simulink model "remote_IAI_rcp"  (R2023a)
settings: Solver=ode1  StartTime=0.0  StopTime=inf  FixedStep=0.02  RelTol=1e-3
undefined symbols (not defined in the file): f, none, videoinput
libraries: simulink x9, instrumentlib x3, imaqlib x1, visionsinks x1
settings Model: Creator=nkobayas  LastModifiedBy=nkobayas

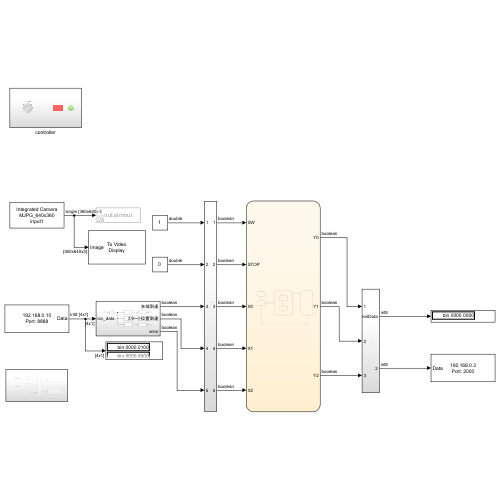
[thumbnail: Simulink's stored preview of the top-level diagram]
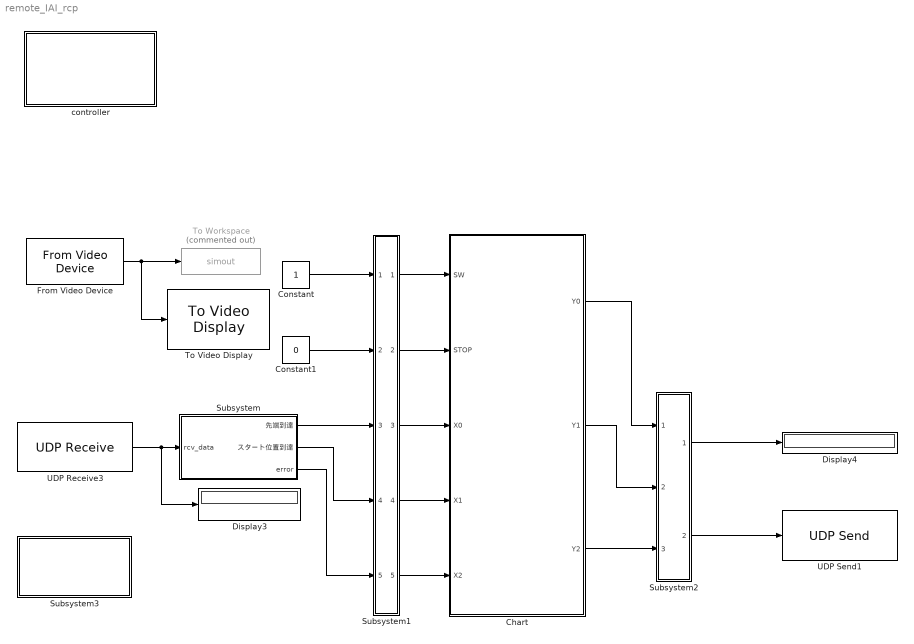
== system remote_IAI_rcp ==
  Chart : Stateflow chart  TreatAsAtomicUnit=on
  Constant : Constant
  Constant1 : Constant  Value=0
  Display3 : Display
      settings: Format=binary (Stored Integer)
  Display4 : Display
      settings: Format=binary (Stored Integer)
  From Video Device : imaqlib/From Video Device  DeviceMenu=winvideo 1 (Integrated Camera)  Device=winvideo 1 (Integrated Camera)  ObjConstructor=videoinput('winvideo', 1)  VideoFormatMenu=MJPG_640x360  VideoFormat=MJPG_640x360  VideoSource=input1  ROIPosition=[0 0 360 640]  EnableHWTrigger=off  TriggerConfiguration=none/none  SampleTime=0.02  OutputPortsMode=One multidimensional signal  DataType=single  CanDoHWTrigger=no  ReturnedColorSpace=rgb  BlockHandle=264.0006  ROIWidth=640  ROIHeight=360  ROIColumn=0  ROIRow=0  EngXMLPath=C:\Program Files\MATLAB\R2023a\toolbox\imaq\imaq\private  DevXMLPath=C:\ProgramData\MATLAB\SupportPackages\R2023a\toolbox\imaq\supportpackages\genericvideo\adaptor\win64  EngLibPath=C:\Program Files\MATLAB\R2023a\toolbox\imaq\imaqblks\imaqmex\win64  ColorSpace=rgb  BayerSensorAlignment=grbg  ImaqMode=off
  Subsystem : Subsystem
  Subsystem1 : Subsystem
  Subsystem2 : Subsystem
  Subsystem3 : Subsystem
  To Video Display : visionsinks/To Video Display  windowSizeMode=Normal  openAtMdlStart=on  fullScreen=off  videoWindowX=26  videoWindowY=640  saveWindowSize=off  videoWindowWidth=640  videoWindowHeight=360  inputColorFormat=RGB  inputType=Obsolete  imagePorts=One multidimensional signal  OutputDevice=On-screen video monitor  dataOrg=Column-major  isWindowOpen=off
  To Workspace : ToWorkspace  Commented=on  VariableName=simout  SaveFormat=Timeseries  SampleTime=-1
  UDP Receive3 : instrumentlib/UDP Receive  LocalAddress=192.168.0.10  LocalPort=8888  EnablePortSharing=on  Host=192.168.0.3  Port=2000  GetLatestData=on  DataSize=4  DataType=int8  ASCIIFormatting=%f,  Terminator=LF  CustomTerminator=10  ByteOrder=little-endian  EnableBlockingMode=on  Timeout=10  SampleTime=0.02  SimulateUsing=Interpreted execution
  UDP Send1 : instrumentlib/UDP Send  Host=192.168.0.3  Port=2000  LocalAddress=192.168.0.10  LocalPort=8888  EnablePortSharing=on  OutputDatagramPacketSize=8  ByteOrder=little-endian  EnableBlockingMode=off  SimulateUsing=Interpreted execution
  controller : Subsystem
  wires:
  Chart/3(Y2) -> Subsystem2/3(In3)
  Chart/2(Y1) -> Subsystem2/2(In2)
  Chart/1(Y0) -> Subsystem2/1(In1)
  Subsystem2/2(Out2) -> UDP Send1/1
  Subsystem2/1(serverSendData) -> Display4/1
  UDP Receive3/1 -> Subsystem/1(rcv_data), Display3/1
  Constant/1 -> Subsystem1/1(In1)
  Constant1/1 -> Subsystem1/2(In2)
  Subsystem/1(先端到達) -> Subsystem1/3(In3)
  Subsystem/2(スタート位置到達) -> Subsystem1/4(In4)
  Subsystem/3(error) -> Subsystem1/5(In5)
  Subsystem1/1(Out1) -> Chart/1(SW)
  Subsystem1/2(Out2) -> Chart/2(STOP)
  Subsystem1/3(Out3) -> Chart/3(X0)
  Subsystem1/4(Out4) -> Chart/4(X1)
  Subsystem1/5(Out5) -> Chart/5(X2)
  From Video Device/1 -> To Video Display/1, To Workspace/1

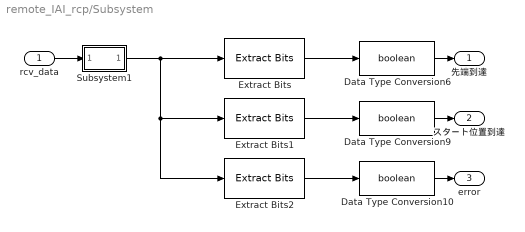
== system remote_IAI_rcp/Subsystem ==
  rcv_data : Inport
  Data Type Conversion10 : DataTypeConversion  OutDataTypeStr=boolean  SaturateOnIntegerOverflow=off  RndMeth=Floor
  Data Type Conversion6 : DataTypeConversion  OutDataTypeStr=boolean  SaturateOnIntegerOverflow=off  RndMeth=Floor
  Data Type Conversion9 : DataTypeConversion  OutDataTypeStr=boolean  SaturateOnIntegerOverflow=off  RndMeth=Floor
  Extract Bits : simulink/Logic and Bit Operations/Extract Bits  bitsToExtract=Range of bits  numBits=8  bitIdxRange=2  outScalingMode=Treat bit field as an integer
  Extract Bits1 : simulink/Logic and Bit Operations/Extract Bits  bitsToExtract=Range of bits  numBits=8  bitIdxRange=0  outScalingMode=Treat bit field as an integer
  Extract Bits2 : simulink/Logic and Bit Operations/Extract Bits  bitsToExtract=Range of bits  numBits=8  bitIdxRange=4  outScalingMode=Treat bit field as an integer
  Subsystem1 : Subsystem
  先端到達 : Outport
  スタート位置到達 : Outport  Port=2
  error : Outport  Port=3
  wires:
  Data Type Conversion6/1 -> 先端到達/1
  Subsystem1/1(rcv_data) -> Extract Bits2/1, Extract Bits1/1, Extract Bits/1
  Extract Bits/1 -> Data Type Conversion6/1
  Extract Bits2/1 -> Data Type Conversion10/1
  Extract Bits1/1 -> Data Type Conversion9/1
  Data Type Conversion10/1 -> error/1
  Data Type Conversion9/1 -> スタート位置到達/1
  rcv_data/1 -> Subsystem1/1(In1)

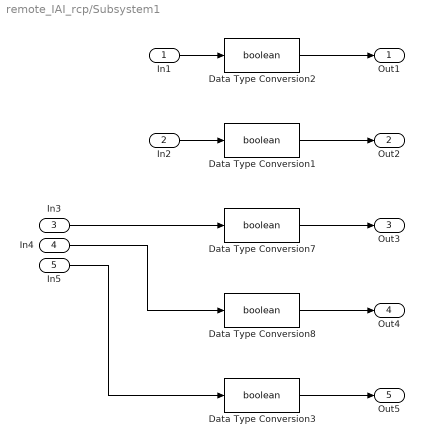
== system remote_IAI_rcp/Subsystem1 ==
  In1 : Inport
  In2 : Inport  Port=2
  In3 : Inport  Port=3
  In4 : Inport  Port=4
  In5 : Inport  Port=5
  Data Type Conversion{1..3,7..8} (5 alike) : DataTypeConversion  OutDataTypeStr=boolean  SaturateOnIntegerOverflow=off  RndMeth=Floor
  Out1 : Outport
  Out2 : Outport  Port=2
  Out3 : Outport  Port=3
  Out4 : Outport  Port=4
  Out5 : Outport  Port=5
  wires:
  Data Type Conversion3/1 -> Out5/1
  In5/1 -> Data Type Conversion3/1
  Data Type Conversion7/1 -> Out3/1
  In2/1 -> Data Type Conversion1/1
  Data Type Conversion8/1 -> Out4/1
  In1/1 -> Data Type Conversion2/1
  In3/1 -> Data Type Conversion7/1
  In4/1 -> Data Type Conversion8/1
  Data Type Conversion1/1 -> Out2/1
  Data Type Conversion2/1 -> Out1/1

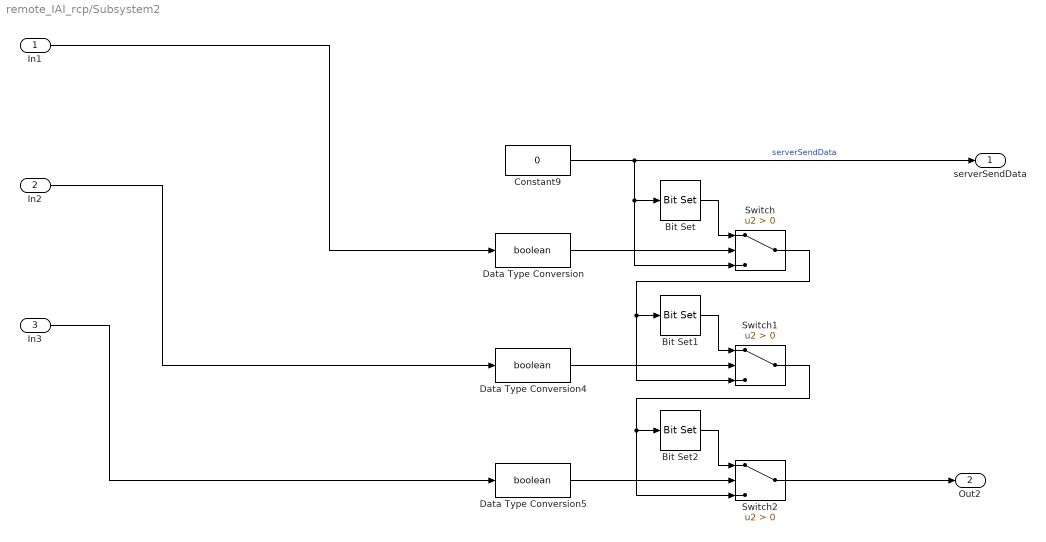
== system remote_IAI_rcp/Subsystem2 ==
  In1 : Inport
  In2 : Inport  Port=2
  In3 : Inport  Port=3
  Bit Set : simulink/Logic and Bit Operations/Bit Set  iBit=0
  Bit Set1 : simulink/Logic and Bit Operations/Bit Set  iBit=1
  Bit Set2 : simulink/Logic and Bit Operations/Bit Set  iBit=2
  Constant9 : Constant  Value=0  OutDataTypeStr=int8
  Data Type Conversion : DataTypeConversion  OutDataTypeStr=boolean  SaturateOnIntegerOverflow=off  RndMeth=Floor
  Data Type Conversion4 : DataTypeConversion  OutDataTypeStr=boolean  SaturateOnIntegerOverflow=off  RndMeth=Floor
  Data Type Conversion5 : DataTypeConversion  OutDataTypeStr=boolean  SaturateOnIntegerOverflow=off  RndMeth=Floor
  Switch : Switch  Criteria=u2 > Threshold  SaturateOnIntegerOverflow=off  InputSameDT=off
  Switch1 : Switch  Criteria=u2 > Threshold  SaturateOnIntegerOverflow=off  InputSameDT=off
  Switch2 : Switch  Criteria=u2 > Threshold  SaturateOnIntegerOverflow=off  InputSameDT=off
  serverSendData : Outport
  Out2 : Outport  Port=2
  wires:
  In1/1 -> Data Type Conversion/1
  In2/1 -> Data Type Conversion4/1
  Bit Set2/1 -> Switch2/1
  Bit Set1/1 -> Switch1/1
  Switch/1 -> Bit Set1/1, Switch1/3
  Switch2/1 -> Out2/1
  Data Type Conversion5/1 -> Switch2/2
  Switch1/1 -> Bit Set2/1, Switch2/3
  In3/1 -> Data Type Conversion5/1
  Bit Set/1 -> Switch/1
  Data Type Conversion/1 -> Switch/2
  Constant9/1 -> Bit Set/1, Switch/3, serverSendData/1  "serverSendData"
  Data Type Conversion4/1 -> Switch1/2

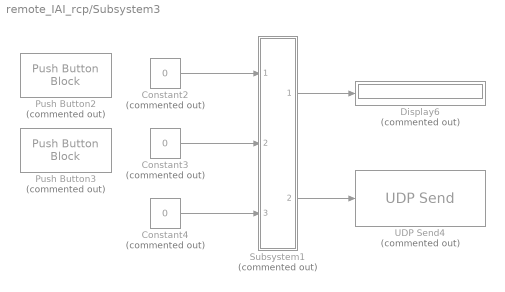
== system remote_IAI_rcp/Subsystem3 ==
  Constant2 : Constant  Commented=on  Value=0
  Constant3 : Constant  Commented=on  Value=0
  Constant4 : Constant  Commented=on  Value=0
  Display6 : Display  Commented=on
      settings: Format=binary (Stored Integer)
  Push Button2 : PushButtonBlock  Commented=on  ButtonText=ON_F  OffValue=0.000000
  Push Button3 : PushButtonBlock  Commented=on  ButtonText=ON_B  OffValue=0.000000
  Subsystem1 : Subsystem  Commented=on
  UDP Send4 : instrumentlib/UDP Send  Commented=on  Host=192.168.0.3  Port=2000  LocalAddress=192.168.0.10  LocalPort=8888  EnablePortSharing=on  OutputDatagramPacketSize=8  ByteOrder=little-endian  EnableBlockingMode=off  SimulateUsing=Interpreted execution
  wires:
  Subsystem1/1(serverSendData) -> Display6/1
  Constant2/1 -> Subsystem1/1(In1)
  Constant3/1 -> Subsystem1/2(In2)
  Subsystem1/2(Out2) -> UDP Send4/1
  Constant4/1 -> Subsystem1/3(In3)

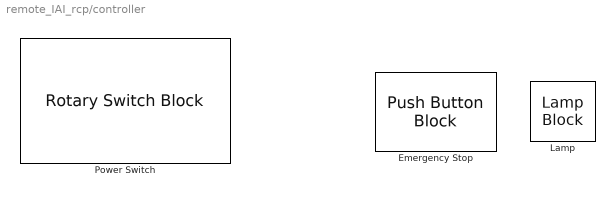
== system remote_IAI_rcp/controller ==
  Emergency Stop : PushButtonBlock  ButtonText=STOP  ButtonType=Latch  OffValue=0.000000
  Lamp : LampBlock  LabelPosition=Hide
  Power Switch : RotarySwitchBlock
      settings: Values={{'OFF', 'ON'}, [0 1]}

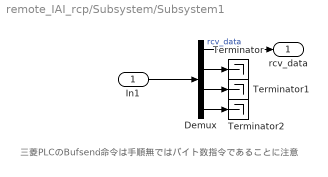
== system remote_IAI_rcp/Subsystem/Subsystem1 ==
  note: 三菱PLCのBufsend命令は手順無ではバイト数指令であることに注意
  In1 : Inport
  Demux : Demux
  Terminator : Terminator
  Terminator1 : Terminator
  Terminator2 : Terminator
  rcv_data : Outport
  wires:
  In1/1 -> Demux/1
  Demux/1 -> rcv_data/1  "rcv_data"
  Demux/2 -> Terminator/1
  Demux/3 -> Terminator1/1
  Demux/4 -> Terminator2/1

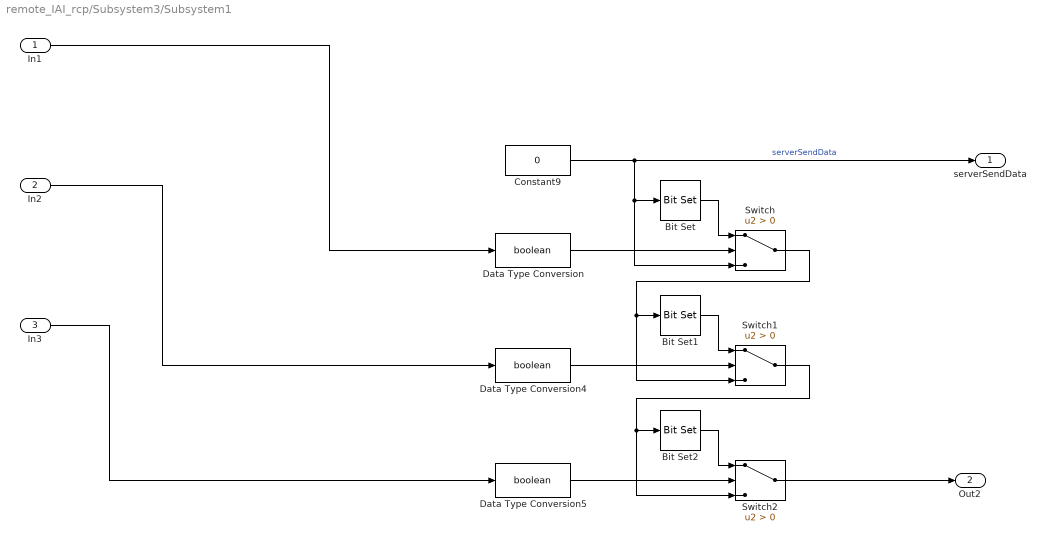
== system remote_IAI_rcp/Subsystem3/Subsystem1 ==
  In1 : Inport
  In2 : Inport  Port=2
  In3 : Inport  Port=3
  Bit Set : simulink/Logic and Bit Operations/Bit Set  iBit=0
  Bit Set1 : simulink/Logic and Bit Operations/Bit Set  iBit=1
  Bit Set2 : simulink/Logic and Bit Operations/Bit Set  iBit=2
  Constant9 : Constant  Value=0  OutDataTypeStr=int8
  Data Type Conversion : DataTypeConversion  OutDataTypeStr=boolean  SaturateOnIntegerOverflow=off  RndMeth=Floor
  Data Type Conversion4 : DataTypeConversion  OutDataTypeStr=boolean  SaturateOnIntegerOverflow=off  RndMeth=Floor
  Data Type Conversion5 : DataTypeConversion  OutDataTypeStr=boolean  SaturateOnIntegerOverflow=off  RndMeth=Floor
  Switch : Switch  Criteria=u2 > Threshold  SaturateOnIntegerOverflow=off  InputSameDT=off
  Switch1 : Switch  Criteria=u2 > Threshold  SaturateOnIntegerOverflow=off  InputSameDT=off
  Switch2 : Switch  Criteria=u2 > Threshold  SaturateOnIntegerOverflow=off  InputSameDT=off
  serverSendData : Outport
  Out2 : Outport  Port=2
  wires:
  Data Type Conversion4/1 -> Switch1/2
  Constant9/1 -> serverSendData/1, Switch/3, Bit Set/1  "serverSendData"
  Data Type Conversion/1 -> Switch/2
  Bit Set/1 -> Switch/1
  In3/1 -> Data Type Conversion5/1
  Switch1/1 -> Switch2/3, Bit Set2/1
  Data Type Conversion5/1 -> Switch2/2
  Switch2/1 -> Out2/1
  Switch/1 -> Switch1/3, Bit Set1/1
  Bit Set1/1 -> Switch1/1
  Bit Set2/1 -> Switch2/1
  In2/1 -> Data Type Conversion4/1
  In1/1 -> Data Type Conversion/1

== stateflow chart remote_IAI_rcp/Chart ==
  state Moving
    state Foward
      Y0 = true;
      Y1 = false;
      Y2 = false;
    state Back
      Y0 = false;
      Y1 = true;
      Y2 = false;
    (default) -> Foward
    Foward -> Back : [(X0 == true)&&...
        | after(3,sec)]
    Back -> Foward : [(X1 == true)&&...
        | after(3,sec)]
  state Error
    Y0 = false;
    Y1 = false;
    Y2 = false;
  state Init
    Y0 = false;
    Y1 = false;
    Y2 = false;
  state Wait
    Y0 = false;
    Y1 = true;
    Y2 = true;
  (default) -> Init
  Moving -> Error [order 1] : [STOP==true||...
      | X2==true]
  Init -> Wait : after(1,sec)
  Wait -> Moving : [SW==true&&...
      | after(5,sec)]
  Moving -> Wait [order 2] : [SW==false&&...
      | after(3,sec)]
  (junction 35) -> Wait
  Error -> (junction 33) : [STOP==false&&...
      | X2==false]
  (junction 33) -> (junction 35)
  data: SW input; STOP input; Y0 output; Y1 output; Y2 output; X0 input; X1 input; X2 input
